simulink model "deteccao_erro_2014"  (R2014b)
settings: Solver=ode45  StartTime=72.6  StopTime=72.8  FixedStep=Ts  MaxStep=1e-7  RelTol=1e-5  AbsTol=1e-5
undefined symbols (not defined in the file or in its folder): C, L, sigbuilder_block, Ts
libraries: powerlib x59, dsparch4 x12, simulink x6, sps_avr x1, powerlib_meascontrol x1
(part 2 of 2)

== system deteccao_erro_2014/EHA1/DSP/Subsystem ==
  Vabc' : Inport
  Iabc_L : Inport  Port=2
  Demux : Demux  Outputs=3
  Demux6 : Demux  Outputs=3
  Gain1 : Gain  Gain=sqrt(2/3)
  Gain2 : Gain  Gain=sqrt(2/3)
  Gain3 : Gain  Gain=[1/sqrt(2), 1/sqrt(2), 1/sqrt(2); 1, -1/2, -1/2; 0, sqrt(3)/2, -sqrt(3)/2]  Multiplication=Matrix(K*u)
  Gain4 : Gain  Gain=[1/sqrt(2), 1/sqrt(2), 1/sqrt(2); 1, -1/2, -1/2; 0, sqrt(3)/2, -sqrt(3)/2]  Multiplication=Matrix(K*u)
  Scope15 : Scope  NumInputPorts=2
      settings: YMin=-600~-200  YMax=400~200  SaveName=ScopeData33
  Terminator : Terminator
  Terminator1 : Terminator
  Valpha' : Outport
  Vbeta' : Outport  Port=2
  Ialpha : Outport  Port=3
  Ibeta : Outport  Port=4
  wires:
  Gain1/1 -> Gain3/1
  Gain2/1 -> Gain4/1
  Gain3/1 -> Demux/1, Scope15/1  "Valphabeta0"
  Demux/2 -> Valpha'/1  "Valpha"
  Demux6/2 -> Ialpha/1  "Ialpha"
  Demux/3 -> Vbeta'/1  "Vbeta"
  Demux6/3 -> Ibeta/1  "Ibeta"
  Iabc_L/1 -> Gain2/1
  Vabc'/1 -> Gain1/1
  Gain4/1 -> Demux6/1, Scope15/2  "Ialphabeta0"
  Demux6/1 -> Terminator/1  "I0"
  Demux/1 -> Terminator1/1  "V0"

== system deteccao_erro_2014/EHA1/DSP/Subsystem1 ==
  Valpha' : Inport
  Vbeta' : Inport  Port=2
  Ialpha : Inport  Port=3
  Ibeta : Inport  Port=4
  Add : Sum
  Add10 : Sum
  Add3 : Sum  Inputs=+-
  Add4 : Sum  Inputs=+-
  LPF : dsparch4/Analog Filter Design  method=Butterworth  filttype=Lowpass  N=5  Wlo=2*pi*200  Whi=80  Rp=2  Rs=40
  Product{5..8} (4 alike) : Product
  Scope18 : Scope  NumInputPorts=4
      settings: TimeRange=0.015  YMin=120~175.6~-2050~-2100  YMax=250~177.8~-1400~-1400  SaveName=ScopeData35
  Posc : Outport
  q : Outport  Port=2
  wires:
  Product5/1 -> Add/1
  Product6/1 -> Add/2
  Add/1 -> Add4/2, LPF/1, Scope18/1  "P"
  Product7/1 -> Add3/1
  Product8/1 -> Add3/2
  Add3/1 -> q/1  "q"
  LPF/1 -> Add4/1, Scope18/2  "Pbarra"
  Vbeta'/1 -> Product7/1, Product6/1
  Ialpha/1 -> Product7/2, Product5/2
  Valpha'/1 -> Product8/1, Product5/1
  Ibeta/1 -> Product8/2, Product6/2
  Add10/1 -> Posc/1, Scope18/4  "Posc"
  Add4/1 -> Add10/2  "-Ptil"
  [Ploss1] -> Scope18/3, Add10/1  "Ploss"

== system deteccao_erro_2014/EHA1/DSP/Subsystem2 ==
  Valpha' : Inport
  Vbeta' : Inport  Port=2
  Posc : Inport  Port=3
  q : Inport  Port=4
  Add8 : Sum
  Add9 : Sum  Inputs=+-
  Divide{1..4} (4 alike) : Product  Inputs=***
  Fcn : Fcn  Expr=1/(u(1)^2+u(2)^2)
  Gain : Gain
  Gain5 : Gain  Gain=-1
  Mux : Mux  Inputs=2
  Scope20 : Scope  NumInputPorts=2
      settings: YMin=-8~-1e+12  YMax=8~2e+12  SaveName=ScopeData37
  Ialpha_p : Outport
  Ibeta_p : Outport  Port=2
  wires:
  Mux/1 -> Fcn/1
  Valpha'/1 -> Divide4/1, Mux/1, Divide1/1
  Vbeta'/1 -> Mux/2, Divide2/1, Divide3/1
  Posc/1 -> Gain5/1
  Fcn/1 -> Divide4/3, Divide3/3, Divide2/3, Divide1/3
  q/1 -> Gain/1
  Divide1/1 -> Add8/1
  Divide2/1 -> Add8/2
  Divide3/1 -> Add9/1
  Divide4/1 -> Add9/2
  Add9/1 -> Ibeta_p/1, Scope20/2  "Ibeta^*"
  Add8/1 -> Ialpha_p/1, Scope20/1  "Iaplha^*"
  Gain/1 -> Divide2/2, Divide4/2
  Gain5/1 -> Divide1/2, Divide3/2

== system deteccao_erro_2014/EHA1/DSP/Subsystem3 ==
  Ialpha_p : Inport
  Ibeta_p : Inport  Port=2
  Fcn1 : Fcn  Expr=sqrt(2/3)*u(1)
  Fcn2 : Fcn  Expr=sqrt(2/3)*(-1/2*u(1)+sqrt(3)/2*u(2))
  Fcn3 : Fcn  Expr=sqrt(2/3)*(-1/2*u(1)-sqrt(3)/2*u(2))
  Mux2 : Mux  Inputs=2
  Mux3 : Mux  Inputs=2
  Mux5 : Mux  Inputs=2
  Scope14 : Scope  NumInputPorts=3
      settings: TimeRange=0.08  YMin=-4~-4.5~-2  YMax=4.5~4~4.5  SaveName=ScopeData32
  Ia_C : Outport
  Ib_C : Outport  Port=2
  Ic_C : Outport  Port=3
  wires:
  Ibeta_p/1 -> Mux2/2, Mux3/2, Mux5/2
  Ialpha_p/1 -> Mux5/1, Mux2/1, Mux3/1
  Mux2/1 -> Fcn1/1
  Fcn1/1 -> Ia_C/1, Scope14/1  "Ia_C"
  Mux3/1 -> Fcn2/1
  Fcn2/1 -> Ib_C/1, Scope14/2  "Ib_C"
  Mux5/1 -> Fcn3/1
  Fcn3/1 -> Scope14/3, Ic_C/1  "Ic_C"

== system deteccao_erro_2014/EHA1/DSP/TCT ==
  Va : Inport
  Vb : Inport  Port=2
  Vc : Inport  Port=3
  Demux7 : Demux  Outputs=3
  Gain1 : Gain  Gain=sqrt(2/3)
  Gain3 : Gain  Gain=[1/sqrt(2), 1/sqrt(2), 1/sqrt(2); 1, -1/2, -1/2; 0, sqrt(3)/2, -sqrt(3)/2]  Multiplication=Matrix(K*u)
  Mux2 : Mux  Inputs=3
  valpha : Outport
  vbeta : Outport  Port=2
  wires:
  Gain3/1 -> Demux7/1  "Valphabeta0"
  Gain1/1 -> Gain3/1
  Mux2/1 -> Gain1/1
  Va/1 -> Mux2/1
  Vb/1 -> Mux2/2
  Vc/1 -> Mux2/3
  Demux7/2 -> valpha/1
  Demux7/3 -> vbeta/1

== system deteccao_erro_2014/EHA1/DSP/Transformada Inversa de Clarke ==
  valpha' : Inport
  vbeta' : Inport  Port=2
  Demux6 : Demux  Outputs=3
  Fcn10 : Fcn  Expr=sqrt(2/3)*(-1/2*u(1)+sqrt(3)/2*u(2))
  Fcn11 : Fcn  Expr=sqrt(2/3)*(-1/2*u(1)-sqrt(3)/2*u(2))
  Fcn9 : Fcn  Expr=sqrt(2/3)*(u(1) + 0*u(2))
  Mux{3,5,8..9} (4 alike) : Mux  Inputs=2
  Scope23 : Scope  NumInputPorts=3
      settings: YMin=-200~-200~-200  YMax=200~200~200  SaveName=ScopeData28
  va' : Outport
  vb' : Outport  Port=2
  vc' : Outport  Port=3
  wires:
  Fcn10/1 -> vb'/1, Scope23/2  "vb'"
  Demux6/1 -> Mux9/1
  valpha'/1 -> Mux5/1, Mux8/1, Mux3/1
  vbeta'/1 -> Mux3/2, Mux5/2, Mux8/2
  Mux5/1 -> Fcn10/1
  Mux3/1 -> Fcn9/1
  Fcn11/1 -> vc'/1, Scope23/3  "vc'"
  Fcn9/1 -> va'/1, Mux9/2  "va'"
  Mux8/1 -> Fcn11/1
  [Vabc_S] -> Demux6/1
  Mux9/1 -> Scope23/1

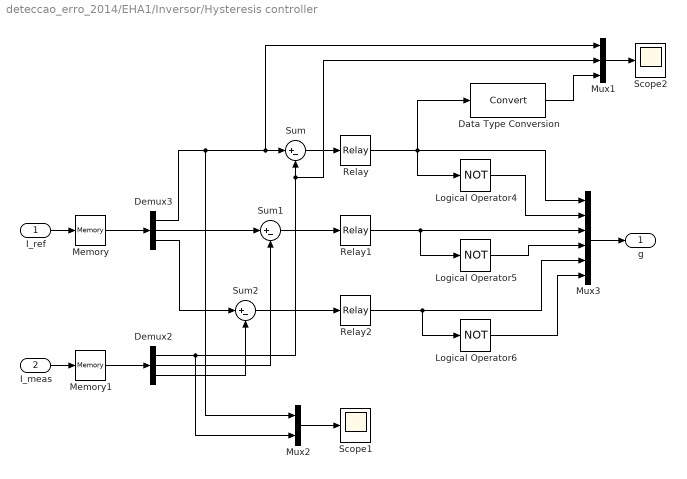
== system deteccao_erro_2014/EHA1/Inversor/Hysteresis controller ==
  I_ref : Inport
  I_meas : Inport  Port=2
  Data Type Conversion : DataTypeConversion
  Demux2 : Demux  Outputs=3
  Demux3 : Demux  Outputs=3
  Logical Operator4 : Logic  Operator=NOT  AllPortsSameDT=off  OutDataTypeStr=boolean
  Logical Operator5 : Logic  Operator=NOT  AllPortsSameDT=off  OutDataTypeStr=boolean
  Logical Operator6 : Logic  Operator=NOT  AllPortsSameDT=off  OutDataTypeStr=boolean
  Memory : Memory
  Memory1 : Memory
  Mux1 : Mux  Inputs=3
  Mux2 : Mux  Inputs=2
  Mux3 : Mux  Inputs=6
  Relay : Relay  OnSwitchValue=0.05  OffSwitchValue=-0.05  OutDataTypeStr=Inherit: Inherit via back propagation
  Relay1 : Relay  OnSwitchValue=0.05  OffSwitchValue=-0.05  OutDataTypeStr=Inherit: Inherit via back propagation
  Relay2 : Relay  OnSwitchValue=0.05  OffSwitchValue=-0.05  OutDataTypeStr=Inherit: Inherit via back propagation
  Scope1 : Scope
      settings: YMin=-3.75e+12  YMax=2.5e+11  SaveName=ScopeData30
  Scope2 : Scope
      settings: YMin=-4.5  YMax=5.5  SaveName=ScopeData6
  Sum : Sum  Inputs=|+-
  Sum1 : Sum  Inputs=|+-
  Sum2 : Sum  Inputs=|+-
  g : Outport
  wires:
  I_ref/1 -> Memory/1
  I_meas/1 -> Memory1/1
  Relay1/1 -> Logical Operator5/1, Mux3/3
  Demux3/1 -> Mux1/1, Sum/1, Mux2/1
  Logical Operator4/1 -> Mux3/2
  Logical Operator5/1 -> Mux3/4
  Logical Operator6/1 -> Mux3/6
  Mux3/1 -> g/1
  Demux2/1 -> Mux2/2, Mux1/2, Sum/2
  Memory/1 -> Demux3/1
  Memory1/1 -> Demux2/1
  Mux2/1 -> Scope1/1
  Sum/1 -> Relay/1
  Relay/1 -> Data Type Conversion/1, Mux3/1, Logical Operator4/1
  Demux3/2 -> Sum1/1
  Demux2/2 -> Sum1/2
  Sum1/1 -> Relay1/1
  Demux3/3 -> Sum2/1
  Sum2/1 -> Relay2/1
  Demux2/3 -> Sum2/2
  Relay2/1 -> Mux3/5, Logical Operator6/1
  Mux1/1 -> Scope2/1
  Data Type Conversion/1 -> Mux1/3

== system deteccao_erro_2014/EHA1/Inversor/PI controller ==
  Vdc : Inport
  Constant : Constant  Value=620
  LPF : dsparch4/Analog Filter Design  method=Butterworth  filttype=Lowpass  N=5  Wlo=2*pi*200  Whi=80  Rp=2  Rs=40
  PID Controller : simulink/Continuous/PID Controller  Controller=PI  TimeDomain=Continuous-time  SampleTime=-1  IntegratorMethod=Forward Euler  FilterMethod=Forward Euler  Form=Parallel  P=5  I=7  D=0  N=100  InitialConditionSource=internal  InitialConditionForIntegrator=0  InitialConditionForFilter=0  ExternalReset=none  LimitOutput=off  UpperSaturationLimit=inf  LowerSaturationLimit=-inf  LinearizeAsGain=on  AntiWindupMode=none  Kb=1  TrackingMode=off  Kt=1  PParamMin=[]  PParamMax=[]  IParamMin=[]  IParamMax=[]  DParamMin=[]  DParamMax=[]  NParamMin=[]  NParamMax=[]  KbParamMin=[]  KbParamMax=[]  KtParamMin=[]  KtParamMax=[]  POutMin=[]  POutMax=[]  IOutMin=[]  IOutMax=[]  DOutMin=[]  DOutMax=[]  NOutMin=[]  NOutMax=[]  KbOutMin=[]  KbOutMax=[]  KtOutMin=[]  KtOutMax=[]  IntegratorOutMin=[]  IntegratorOutMax=[]  FilterOutMin=[]  FilterOutMax=[]  SumOutMin=[]  SumOutMax=[]  SumI1OutMin=[]  SumI1OutMax=[]  SumI2OutMin=[]  SumI2OutMax=[]  SumI3OutMin=[]  SumI3OutMax=[]  SumDOutMin=[]  SumDOutMax=[]  SaturationOutMin=[]  SaturationOutMax=[]  IntegratorContinuousStateAttributes=''  IntegratorStateMustResolveToSignalObject=off  IntegratorRTWStateStorageClass=Auto  FilterContinuousStateAttributes=''  FilterStateMustResolveToSignalObject=off  FilterRTWStateStorageClass=Auto  DifferentiatorICPrevScaledInput=0  DifferentiatorOutMin=[]  DifferentiatorOutMax=[]  UseFilter=on
  Scope : Scope  NumInputPorts=3
      settings: TimeRange=0.015  YMin=-5~-5~-5  YMax=5~5~5  SaveName=ScopeData18
  Signal Builder : Subsystem  Tag=STV Subsys  LoadFcn=sigbuilder_block('load');  StartFcn=sigbuilder_block('start');  StopFcn=sigbuilder_block('stop');  ClipboardFcn=sigbuilder_block('clipboard');  mask(Sigbuilder block){}
      mask help: Simulink:masks:SigbuilderBlock_MD
      mask init:
      | if ~strcmp(get_param(bdroot(gcbh),'SimulationStatus'),'stopped') tuvar = sigbuilder_block('maskInit'); end
      settings: CopyFcn=sigbuilder_block('copy');  DeleteFcn=sigbuilder_block('delete');  ModelCloseFcn=sigbuilder_block('modelClose');  PreSaveFcn=sigbuilder_block('preSave');  PauseFcn=sigbuilder_block('pause');  ContinueFcn=sigbuilder_block('continue');  NameChangeFcn=sigbuilder_block('namechange');  OpenFcn=sigbuilder_block('open',[437.6 199.2 550.4 400 ]);  CloseFcn=sigbuilder_block('close');
      mask Display: plot(0, 0, 100, 100,[2, 2, 32, 32, 2], [68, 8, 8, 68, 68],[32, 2], [38, 38], [32, 19, 2],[53, 60, 44], [32, 17, 17, 2],[16, 16, 31, 31]);txt = getActiveGroup(gcbh);text(2, 100, txt,'verticalAlignment', 'top');
  Sum : Sum  Inputs=|-+
  Ploss : Outport
  wires:
  Vdc/1 -> Scope/1, Sum/1  "Vdc"
  Sum/1 -> LPF/1, Scope/2  "Vdc-step"
  PID Controller/1 -> Scope/3, Ploss/1  "Ploss"
  LPF/1 -> PID Controller/1
  Signal Builder/1(Signal 2) -> Sum/2

== system deteccao_erro_2014/EHA2/DSP/Calculo de potência Instantânea ==
  Ialpha' : Inport
  Ibeta' : Inport  Port=2
  valpha : Inport  Port=3
  vbeta : Inport  Port=4
  Fcn5 : Fcn  Expr=u(1)*u(3)+u(2)*u(4)
  Fcn6 : Fcn  Expr=u(2)*u(3)-u(1)*u(4)
  LPF : dsparch4/Analog Filter Design  method=Butterworth  filttype=Lowpass  N=5  Wlo=2*pi*100  Whi=80  Rp=2  Rs=40
  LPF1 : dsparch4/Analog Filter Design  method=Butterworth  filttype=Lowpass  N=5  Wlo=2*pi*100  Whi=80  Rp=2  Rs=40
  Mux2 : Mux
  pbarra' : Outport
  qbarra' : Outport  Port=2
  wires:
  Ibeta'/1 -> Mux2/4
  Ialpha'/1 -> Mux2/3
  LPF1/1 -> qbarra'/1
  LPF/1 -> pbarra'/1
  Mux2/1 -> Fcn6/1, Fcn5/1
  Fcn6/1 -> LPF1/1  "q'"
  Fcn5/1 -> LPF/1  "p'"
  vbeta/1 -> Mux2/2
  valpha/1 -> Mux2/1

== system deteccao_erro_2014/EHA2/DSP/Cálculo de tensões alpha-beta ==
  Ialpha' : Inport
  Ibeta' : Inport  Port=2
  pbarra' : Inport  Port=3
  qbarra' : Inport  Port=4
  Add8 : Sum
  Divide5 : Product  Inputs=**
  Divide6 : Product  Inputs=**
  Divide8 : Product  Inputs=*/
  Divide9 : Product  Inputs=*/
  Fcn7 : Fcn  Expr=u(3)*u(1)-u(4)*u(2)
  Fcn8 : Fcn  Expr=u(4)*u(1)+u(3)*u(2)
  Gain8 : Gain
  Gain9 : Gain
  Mux6 : Mux
  valpha' : Outport
  vbeta' : Outport  Port=2
  wires:
  pbarra'/1 -> Gain8/1
  Divide5/1 -> Add8/1
  Divide6/1 -> Add8/2
  Gain8/1 -> Mux6/1
  Fcn8/1 -> Divide9/1
  Mux6/1 -> Fcn8/1, Fcn7/1
  qbarra'/1 -> Gain9/1
  Divide8/1 -> valpha'/1
  Fcn7/1 -> Divide8/1
  Gain9/1 -> Mux6/2
  Divide9/1 -> vbeta'/1
  Ibeta'/1 -> Mux6/4, Divide6/1, Divide6/2
  Ialpha'/1 -> Mux6/3, Divide5/1, Divide5/2
  Add8/1 -> Divide9/2, Divide8/2

== system deteccao_erro_2014/EHA2/DSP/PLL ==
  Va : Inport
  Vb : Inport  Port=2
  Vc : Inport  Port=3
  Add10 : Sum
  Add3 : Sum  Inputs=+-
  Add4 : Sum  Inputs=+-
  Fcn1 : Fcn  Expr=sin(u(1))
  Fcn2 : Fcn  Expr=sin(u(1)+2*pi/3)
  Fcn3 : Fcn  Expr=sin(u(1)-pi/2)
  Fcn4 : Fcn  Expr=-cos(u(1)-pi/2)
  Integrator : Integrator
  PID Controller : simulink/Continuous/PID Controller  Controller=PI  TimeDomain=Continuous-time  SampleTime=-1  IntegratorMethod=Forward Euler  FilterMethod=Forward Euler  Form=Parallel  P=30  I=1  D=0  N=100  InitialConditionSource=internal  InitialConditionForIntegrator=0  InitialConditionForFilter=0  ExternalReset=none  LimitOutput=off  UpperSaturationLimit=inf  LowerSaturationLimit=-inf  LinearizeAsGain=on  AntiWindupMode=none  Kb=1  TrackingMode=off  Kt=1  PParamMin=[]  PParamMax=[]  IParamMin=[]  IParamMax=[]  DParamMin=[]  DParamMax=[]  NParamMin=[]  NParamMax=[]  KbParamMin=[]  KbParamMax=[]  KtParamMin=[]  KtParamMax=[]  POutMin=[]  POutMax=[]  IOutMin=[]  IOutMax=[]  DOutMin=[]  DOutMax=[]  NOutMin=[]  NOutMax=[]  KbOutMin=[]  KbOutMax=[]  KtOutMin=[]  KtOutMax=[]  IntegratorOutMin=[]  IntegratorOutMax=[]  FilterOutMin=[]  FilterOutMax=[]  SumOutMin=[]  SumOutMax=[]  SumI1OutMin=[]  SumI1OutMax=[]  SumI2OutMin=[]  SumI2OutMax=[]  SumI3OutMin=[]  SumI3OutMax=[]  SumDOutMin=[]  SumDOutMax=[]  SaturationOutMin=[]  SaturationOutMax=[]  IntegratorContinuousStateAttributes=''  IntegratorStateMustResolveToSignalObject=off  IntegratorRTWStateStorageClass=Auto  FilterContinuousStateAttributes=''  FilterStateMustResolveToSignalObject=off  FilterRTWStateStorageClass=Auto  DifferentiatorICPrevScaledInput=0  DifferentiatorOutMin=[]  DifferentiatorOutMax=[]  UseFilter=on
  Product5 : Product
  Product6 : Product
  Ialpha' : Outport
  Ibeta' : Outport  Port=2
  wires:
  Va/1 -> Add3/1
  Add3/1 -> Product5/2  "Vab"
  Vc/1 -> Add4/1
  Fcn3/1 -> Ialpha'/1
  Fcn1/1 -> Product5/1
  Fcn2/1 -> Product6/2
  Integrator/1 -> Fcn2/1, Fcn4/1, Fcn1/1, Fcn3/1  "wt"
  Product6/1 -> Add10/2
  Vb/1 -> Add4/2, Add3/2
  Product5/1 -> Add10/1
  Add4/1 -> Product6/1  "Vcb"
  PID Controller/1 -> Integrator/1  "w"
  Add10/1 -> PID Controller/1  "P3phi"
  Fcn4/1 -> Ibeta'/1

== system deteccao_erro_2014/EHA2/DSP/Subsystem ==
  Vabc' : Inport
  Iabc_L : Inport  Port=2
  Demux : Demux  Outputs=3
  Demux6 : Demux  Outputs=3
  Gain1 : Gain  Gain=sqrt(2/3)
  Gain2 : Gain  Gain=sqrt(2/3)
  Gain3 : Gain  Gain=[1/sqrt(2), 1/sqrt(2), 1/sqrt(2); 1, -1/2, -1/2; 0, sqrt(3)/2, -sqrt(3)/2]  Multiplication=Matrix(K*u)
  Gain4 : Gain  Gain=[1/sqrt(2), 1/sqrt(2), 1/sqrt(2); 1, -1/2, -1/2; 0, sqrt(3)/2, -sqrt(3)/2]  Multiplication=Matrix(K*u)
  Scope15 : Scope  NumInputPorts=2
      settings: YMin=-600~-200  YMax=400~200  SaveName=ScopeData33
  Terminator : Terminator
  Terminator1 : Terminator
  Valpha' : Outport
  Vbeta' : Outport  Port=2
  Ialpha : Outport  Port=3
  Ibeta : Outport  Port=4
  wires:
  Gain1/1 -> Gain3/1
  Gain2/1 -> Gain4/1
  Gain3/1 -> Demux/1, Scope15/1  "Valphabeta0"
  Demux/2 -> Valpha'/1  "Valpha"
  Demux6/2 -> Ialpha/1  "Ialpha"
  Demux/3 -> Vbeta'/1  "Vbeta"
  Demux6/3 -> Ibeta/1  "Ibeta"
  Iabc_L/1 -> Gain2/1
  Vabc'/1 -> Gain1/1
  Gain4/1 -> Demux6/1, Scope15/2  "Ialphabeta0"
  Demux6/1 -> Terminator/1  "I0"
  Demux/1 -> Terminator1/1  "V0"

== system deteccao_erro_2014/EHA2/DSP/Subsystem1 ==
  Valpha' : Inport
  Vbeta' : Inport  Port=2
  Ialpha : Inport  Port=3
  Ibeta : Inport  Port=4
  Add : Sum
  Add10 : Sum
  Add3 : Sum  Inputs=+-
  Add4 : Sum  Inputs=+-
  LPF : dsparch4/Analog Filter Design  method=Butterworth  filttype=Lowpass  N=5  Wlo=2*pi*200  Whi=80  Rp=2  Rs=40
  Product{5..8} (4 alike) : Product
  Scope18 : Scope  NumInputPorts=4
      settings: TimeRange=0.015  YMin=24750~27050~-494~-2500  YMax=29750~27900~-478~2000  SaveName=ScopeData35
  Posc : Outport
  q : Outport  Port=2
  wires:
  Product5/1 -> Add/1
  Product6/1 -> Add/2
  Add/1 -> Add4/2, LPF/1, Scope18/1  "P"
  Product7/1 -> Add3/1
  Product8/1 -> Add3/2
  Add3/1 -> q/1  "q"
  LPF/1 -> Add4/1, Scope18/2  "Pbarra"
  Vbeta'/1 -> Product7/1, Product6/1
  Ialpha/1 -> Product7/2, Product5/2
  Valpha'/1 -> Product8/1, Product5/1
  Ibeta/1 -> Product8/2, Product6/2
  Add10/1 -> Posc/1, Scope18/4  "Posc"
  Add4/1 -> Add10/2  "-Ptil"
  [Ploss2] -> Scope18/3, Add10/1  "Ploss"

== system deteccao_erro_2014/EHA2/DSP/Subsystem2 ==
  Valpha' : Inport
  Vbeta' : Inport  Port=2
  Posc : Inport  Port=3
  q : Inport  Port=4
  Add8 : Sum
  Add9 : Sum  Inputs=+-
  Divide{1..4} (4 alike) : Product  Inputs=***
  Fcn : Fcn  Expr=1/(u(1)^2+u(2)^2)
  Gain : Gain
  Gain5 : Gain  Gain=-1
  Mux : Mux  Inputs=2
  Scope20 : Scope  NumInputPorts=2
      settings: YMin=-8~-1e+12  YMax=8~2e+12  SaveName=ScopeData37
  Ialpha_p : Outport
  Ibeta_p : Outport  Port=2
  wires:
  Mux/1 -> Fcn/1
  Valpha'/1 -> Divide4/1, Mux/1, Divide1/1
  Vbeta'/1 -> Mux/2, Divide2/1, Divide3/1
  Posc/1 -> Gain5/1
  Fcn/1 -> Divide4/3, Divide3/3, Divide2/3, Divide1/3
  q/1 -> Gain/1
  Divide1/1 -> Add8/1
  Divide2/1 -> Add8/2
  Divide3/1 -> Add9/1
  Divide4/1 -> Add9/2
  Add9/1 -> Ibeta_p/1, Scope20/2  "Ibeta^*"
  Add8/1 -> Ialpha_p/1, Scope20/1  "Iaplha^*"
  Gain/1 -> Divide2/2, Divide4/2
  Gain5/1 -> Divide1/2, Divide3/2

== system deteccao_erro_2014/EHA2/DSP/Subsystem3 ==
  Ialpha_p : Inport
  Ibeta_p : Inport  Port=2
  Fcn1 : Fcn  Expr=sqrt(2/3)*u(1)
  Fcn2 : Fcn  Expr=sqrt(2/3)*(-1/2*u(1)+sqrt(3)/2*u(2))
  Fcn3 : Fcn  Expr=sqrt(2/3)*(-1/2*u(1)-sqrt(3)/2*u(2))
  Mux2 : Mux  Inputs=2
  Mux3 : Mux  Inputs=2
  Mux5 : Mux  Inputs=2
  Scope14 : Scope  NumInputPorts=3
      settings: TimeRange=0.08  YMin=-4~-4.5~-2  YMax=4.5~4~4.5  SaveName=ScopeData32
  Ia_C : Outport
  Ib_C : Outport  Port=2
  Ic_C : Outport  Port=3
  wires:
  Ibeta_p/1 -> Mux2/2, Mux3/2, Mux5/2
  Ialpha_p/1 -> Mux5/1, Mux2/1, Mux3/1
  Mux2/1 -> Fcn1/1
  Fcn1/1 -> Ia_C/1, Scope14/1  "Ia_C"
  Mux3/1 -> Fcn2/1
  Fcn2/1 -> Ib_C/1, Scope14/2  "Ib_C"
  Mux5/1 -> Fcn3/1
  Fcn3/1 -> Scope14/3, Ic_C/1  "Ic_C"

== system deteccao_erro_2014/EHA2/DSP/TCT ==
  Va : Inport
  Vb : Inport  Port=2
  Vc : Inport  Port=3
  Demux7 : Demux  Outputs=3
  Gain1 : Gain  Gain=sqrt(2/3)
  Gain3 : Gain  Gain=[1/sqrt(2), 1/sqrt(2), 1/sqrt(2); 1, -1/2, -1/2; 0, sqrt(3)/2, -sqrt(3)/2]  Multiplication=Matrix(K*u)
  Mux2 : Mux  Inputs=3
  valpha : Outport
  vbeta : Outport  Port=2
  wires:
  Gain3/1 -> Demux7/1  "Valphabeta0"
  Gain1/1 -> Gain3/1
  Mux2/1 -> Gain1/1
  Va/1 -> Mux2/1
  Vb/1 -> Mux2/2
  Vc/1 -> Mux2/3
  Demux7/2 -> valpha/1
  Demux7/3 -> vbeta/1

== system deteccao_erro_2014/EHA2/DSP/Transformada Inversa de Clarke ==
  valpha' : Inport
  vbeta' : Inport  Port=2
  Demux6 : Demux  Outputs=3
  Fcn10 : Fcn  Expr=sqrt(2/3)*(-1/2*u(1)+sqrt(3)/2*u(2))
  Fcn11 : Fcn  Expr=sqrt(2/3)*(-1/2*u(1)-sqrt(3)/2*u(2))
  Fcn9 : Fcn  Expr=sqrt(2/3)*(u(1) + 0*u(2))
  Mux{3,5,8..9} (4 alike) : Mux  Inputs=2
  Scope23 : Scope  NumInputPorts=3
      settings: YMin=-200~-200~-200  YMax=200~200~200  SaveName=ScopeData28
  va' : Outport
  vb' : Outport  Port=2
  vc' : Outport  Port=3
  wires:
  Fcn10/1 -> vb'/1, Scope23/2  "vb'"
  Demux6/1 -> Mux9/1
  valpha'/1 -> Mux5/1, Mux8/1, Mux3/1
  vbeta'/1 -> Mux3/2, Mux5/2, Mux8/2
  Mux5/1 -> Fcn10/1
  Mux3/1 -> Fcn9/1
  Fcn11/1 -> vc'/1, Scope23/3  "vc'"
  Fcn9/1 -> va'/1, Mux9/2  "va'"
  Mux8/1 -> Fcn11/1
  [Vabc_S] -> Demux6/1
  Mux9/1 -> Scope23/1

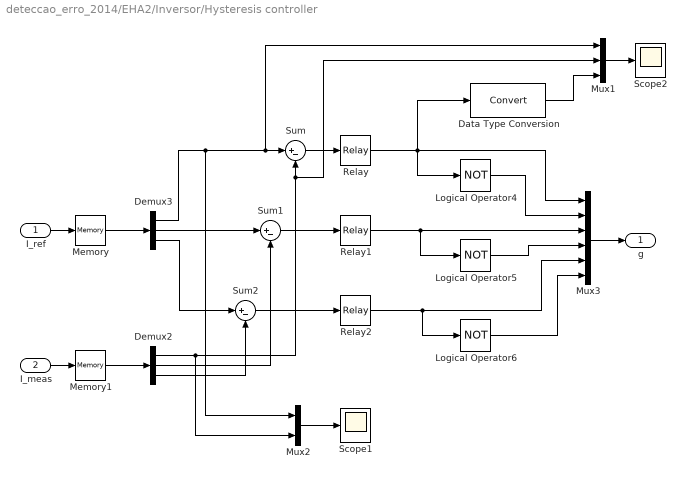
== system deteccao_erro_2014/EHA2/Inversor/Hysteresis controller ==
  I_ref : Inport
  I_meas : Inport  Port=2
  Data Type Conversion : DataTypeConversion
  Demux2 : Demux  Outputs=3
  Demux3 : Demux  Outputs=3
  Logical Operator4 : Logic  Operator=NOT  AllPortsSameDT=off  OutDataTypeStr=boolean
  Logical Operator5 : Logic  Operator=NOT  AllPortsSameDT=off  OutDataTypeStr=boolean
  Logical Operator6 : Logic  Operator=NOT  AllPortsSameDT=off  OutDataTypeStr=boolean
  Memory : Memory
  Memory1 : Memory
  Mux1 : Mux  Inputs=3
  Mux2 : Mux  Inputs=2
  Mux3 : Mux  Inputs=6
  Relay : Relay  OnSwitchValue=0.05  OffSwitchValue=-0.05  OutDataTypeStr=Inherit: Inherit via back propagation
  Relay1 : Relay  OnSwitchValue=0.05  OffSwitchValue=-0.05  OutDataTypeStr=Inherit: Inherit via back propagation
  Relay2 : Relay  OnSwitchValue=0.05  OffSwitchValue=-0.05  OutDataTypeStr=Inherit: Inherit via back propagation
  Scope1 : Scope
      settings: YMin=-3.75e+12  YMax=2.5e+11  SaveName=ScopeData30
  Scope2 : Scope
      settings: YMin=-4.5  YMax=5.5  SaveName=ScopeData6
  Sum : Sum  Inputs=|+-
  Sum1 : Sum  Inputs=|+-
  Sum2 : Sum  Inputs=|+-
  g : Outport
  wires:
  I_ref/1 -> Memory/1
  I_meas/1 -> Memory1/1
  Relay1/1 -> Logical Operator5/1, Mux3/3
  Demux3/1 -> Mux1/1, Sum/1, Mux2/1
  Logical Operator4/1 -> Mux3/2
  Logical Operator5/1 -> Mux3/4
  Logical Operator6/1 -> Mux3/6
  Mux3/1 -> g/1
  Demux2/1 -> Mux2/2, Mux1/2, Sum/2
  Memory/1 -> Demux3/1
  Memory1/1 -> Demux2/1
  Mux2/1 -> Scope1/1
  Sum/1 -> Relay/1
  Relay/1 -> Data Type Conversion/1, Mux3/1, Logical Operator4/1
  Demux3/2 -> Sum1/1
  Demux2/2 -> Sum1/2
  Sum1/1 -> Relay1/1
  Demux3/3 -> Sum2/1
  Sum2/1 -> Relay2/1
  Demux2/3 -> Sum2/2
  Relay2/1 -> Mux3/5, Logical Operator6/1
  Mux1/1 -> Scope2/1
  Data Type Conversion/1 -> Mux1/3

== system deteccao_erro_2014/EHA2/Inversor/PI controller ==
  Vdc : Inport
  Constant : Constant  Value=480
  LPF : dsparch4/Analog Filter Design  method=Butterworth  filttype=Lowpass  N=5  Wlo=2*pi*200  Whi=80  Rp=2  Rs=40
  PID Controller : simulink/Continuous/PID Controller  Controller=PI  TimeDomain=Continuous-time  SampleTime=-1  IntegratorMethod=Forward Euler  FilterMethod=Forward Euler  Form=Parallel  P=5  I=7  D=0  N=100  InitialConditionSource=internal  InitialConditionForIntegrator=0  InitialConditionForFilter=0  ExternalReset=none  LimitOutput=off  UpperSaturationLimit=inf  LowerSaturationLimit=-inf  LinearizeAsGain=on  AntiWindupMode=none  Kb=1  TrackingMode=off  Kt=1  PParamMin=[]  PParamMax=[]  IParamMin=[]  IParamMax=[]  DParamMin=[]  DParamMax=[]  NParamMin=[]  NParamMax=[]  KbParamMin=[]  KbParamMax=[]  KtParamMin=[]  KtParamMax=[]  POutMin=[]  POutMax=[]  IOutMin=[]  IOutMax=[]  DOutMin=[]  DOutMax=[]  NOutMin=[]  NOutMax=[]  KbOutMin=[]  KbOutMax=[]  KtOutMin=[]  KtOutMax=[]  IntegratorOutMin=[]  IntegratorOutMax=[]  FilterOutMin=[]  FilterOutMax=[]  SumOutMin=[]  SumOutMax=[]  SumI1OutMin=[]  SumI1OutMax=[]  SumI2OutMin=[]  SumI2OutMax=[]  SumI3OutMin=[]  SumI3OutMax=[]  SumDOutMin=[]  SumDOutMax=[]  SaturationOutMin=[]  SaturationOutMax=[]  IntegratorContinuousStateAttributes=''  IntegratorStateMustResolveToSignalObject=off  IntegratorRTWStateStorageClass=Auto  FilterContinuousStateAttributes=''  FilterStateMustResolveToSignalObject=off  FilterRTWStateStorageClass=Auto  DifferentiatorICPrevScaledInput=0  DifferentiatorOutMin=[]  DifferentiatorOutMax=[]  UseFilter=on
  Scope : Scope  NumInputPorts=2
      settings: TimeRange=0.015  YMin=-550~450  YMax=25~1025  SaveName=ScopeData15
  Sum : Sum  Inputs=|-+
  Ploss : Outport
  wires:
  Vdc/1 -> Sum/1, Scope/2
  Sum/1 -> LPF/1, Scope/1
  Constant/1 -> Sum/2
  PID Controller/1 -> Ploss/1
  LPF/1 -> PID Controller/1

== system deteccao_erro_2014/EHA3/DSP/Calculo de potência Instantânea ==
  Ialpha' : Inport
  Ibeta' : Inport  Port=2
  valpha : Inport  Port=3
  vbeta : Inport  Port=4
  Fcn5 : Fcn  Expr=u(1)*u(3)+u(2)*u(4)
  Fcn6 : Fcn  Expr=u(2)*u(3)-u(1)*u(4)
  LPF : dsparch4/Analog Filter Design  method=Butterworth  filttype=Lowpass  N=5  Wlo=2*pi*100  Whi=80  Rp=2  Rs=40
  LPF1 : dsparch4/Analog Filter Design  method=Butterworth  filttype=Lowpass  N=5  Wlo=2*pi*100  Whi=80  Rp=2  Rs=40
  Mux2 : Mux
  pbarra' : Outport
  qbarra' : Outport  Port=2
  wires:
  Ibeta'/1 -> Mux2/4
  Ialpha'/1 -> Mux2/3
  LPF1/1 -> qbarra'/1
  LPF/1 -> pbarra'/1
  Mux2/1 -> Fcn6/1, Fcn5/1
  Fcn6/1 -> LPF1/1  "q'"
  Fcn5/1 -> LPF/1  "p'"
  vbeta/1 -> Mux2/2
  valpha/1 -> Mux2/1

== system deteccao_erro_2014/EHA3/DSP/Cálculo de tensões alpha-beta ==
  Ialpha' : Inport
  Ibeta' : Inport  Port=2
  pbarra' : Inport  Port=3
  qbarra' : Inport  Port=4
  Add8 : Sum
  Divide5 : Product  Inputs=**
  Divide6 : Product  Inputs=**
  Divide8 : Product  Inputs=*/
  Divide9 : Product  Inputs=*/
  Fcn7 : Fcn  Expr=u(3)*u(1)-u(4)*u(2)
  Fcn8 : Fcn  Expr=u(4)*u(1)+u(3)*u(2)
  Gain8 : Gain
  Gain9 : Gain
  Mux6 : Mux
  valpha' : Outport
  vbeta' : Outport  Port=2
  wires:
  pbarra'/1 -> Gain8/1
  Divide5/1 -> Add8/1
  Divide6/1 -> Add8/2
  Gain8/1 -> Mux6/1
  Fcn8/1 -> Divide9/1
  Mux6/1 -> Fcn8/1, Fcn7/1
  qbarra'/1 -> Gain9/1
  Divide8/1 -> valpha'/1
  Fcn7/1 -> Divide8/1
  Gain9/1 -> Mux6/2
  Divide9/1 -> vbeta'/1
  Ibeta'/1 -> Mux6/4, Divide6/1, Divide6/2
  Ialpha'/1 -> Mux6/3, Divide5/1, Divide5/2
  Add8/1 -> Divide9/2, Divide8/2

== system deteccao_erro_2014/EHA3/DSP/PLL ==
  Va : Inport
  Vb : Inport  Port=2
  Vc : Inport  Port=3
  Add10 : Sum
  Add3 : Sum  Inputs=+-
  Add4 : Sum  Inputs=+-
  Fcn1 : Fcn  Expr=sin(u(1))
  Fcn2 : Fcn  Expr=sin(u(1)+2*pi/3)
  Fcn3 : Fcn  Expr=sin(u(1)-pi/2)
  Fcn4 : Fcn  Expr=-cos(u(1)-pi/2)
  Integrator : Integrator
  PID Controller : simulink/Continuous/PID Controller  Controller=PI  TimeDomain=Continuous-time  SampleTime=-1  IntegratorMethod=Forward Euler  FilterMethod=Forward Euler  Form=Parallel  P=30  I=1  D=0  N=100  InitialConditionSource=internal  InitialConditionForIntegrator=0  InitialConditionForFilter=0  ExternalReset=none  LimitOutput=off  UpperSaturationLimit=inf  LowerSaturationLimit=-inf  LinearizeAsGain=on  AntiWindupMode=none  Kb=1  TrackingMode=off  Kt=1  PParamMin=[]  PParamMax=[]  IParamMin=[]  IParamMax=[]  DParamMin=[]  DParamMax=[]  NParamMin=[]  NParamMax=[]  KbParamMin=[]  KbParamMax=[]  KtParamMin=[]  KtParamMax=[]  POutMin=[]  POutMax=[]  IOutMin=[]  IOutMax=[]  DOutMin=[]  DOutMax=[]  NOutMin=[]  NOutMax=[]  KbOutMin=[]  KbOutMax=[]  KtOutMin=[]  KtOutMax=[]  IntegratorOutMin=[]  IntegratorOutMax=[]  FilterOutMin=[]  FilterOutMax=[]  SumOutMin=[]  SumOutMax=[]  SumI1OutMin=[]  SumI1OutMax=[]  SumI2OutMin=[]  SumI2OutMax=[]  SumI3OutMin=[]  SumI3OutMax=[]  SumDOutMin=[]  SumDOutMax=[]  SaturationOutMin=[]  SaturationOutMax=[]  IntegratorContinuousStateAttributes=''  IntegratorStateMustResolveToSignalObject=off  IntegratorRTWStateStorageClass=Auto  FilterContinuousStateAttributes=''  FilterStateMustResolveToSignalObject=off  FilterRTWStateStorageClass=Auto  DifferentiatorICPrevScaledInput=0  DifferentiatorOutMin=[]  DifferentiatorOutMax=[]  UseFilter=on
  Product5 : Product
  Product6 : Product
  Ialpha' : Outport
  Ibeta' : Outport  Port=2
  wires:
  Va/1 -> Add3/1
  Add3/1 -> Product5/2  "Vab"
  Vc/1 -> Add4/1
  Fcn3/1 -> Ialpha'/1
  Fcn1/1 -> Product5/1
  Fcn2/1 -> Product6/2
  Integrator/1 -> Fcn2/1, Fcn4/1, Fcn1/1, Fcn3/1  "wt"
  Product6/1 -> Add10/2
  Vb/1 -> Add4/2, Add3/2
  Product5/1 -> Add10/1
  Add4/1 -> Product6/1  "Vcb"
  PID Controller/1 -> Integrator/1  "w"
  Add10/1 -> PID Controller/1  "P3phi"
  Fcn4/1 -> Ibeta'/1

== system deteccao_erro_2014/EHA3/DSP/Subsystem ==
  Vabc' : Inport
  Iabc_L : Inport  Port=2
  Demux : Demux  Outputs=3
  Demux6 : Demux  Outputs=3
  Gain1 : Gain  Gain=sqrt(2/3)
  Gain2 : Gain  Gain=sqrt(2/3)
  Gain3 : Gain  Gain=[1/sqrt(2), 1/sqrt(2), 1/sqrt(2); 1, -1/2, -1/2; 0, sqrt(3)/2, -sqrt(3)/2]  Multiplication=Matrix(K*u)
  Gain4 : Gain  Gain=[1/sqrt(2), 1/sqrt(2), 1/sqrt(2); 1, -1/2, -1/2; 0, sqrt(3)/2, -sqrt(3)/2]  Multiplication=Matrix(K*u)
  Scope15 : Scope  NumInputPorts=2
      settings: YMin=-600~-200  YMax=400~200  SaveName=ScopeData33
  Terminator : Terminator
  Terminator1 : Terminator
  Valpha' : Outport
  Vbeta' : Outport  Port=2
  Ialpha : Outport  Port=3
  Ibeta : Outport  Port=4
  wires:
  Gain1/1 -> Gain3/1
  Gain2/1 -> Gain4/1
  Gain3/1 -> Demux/1, Scope15/1  "Valphabeta0"
  Demux/2 -> Valpha'/1  "Valpha"
  Demux6/2 -> Ialpha/1  "Ialpha"
  Demux/3 -> Vbeta'/1  "Vbeta"
  Demux6/3 -> Ibeta/1  "Ibeta"
  Iabc_L/1 -> Gain2/1
  Vabc'/1 -> Gain1/1
  Gain4/1 -> Demux6/1, Scope15/2  "Ialphabeta0"
  Demux6/1 -> Terminator/1  "I0"
  Demux/1 -> Terminator1/1  "V0"

== system deteccao_erro_2014/EHA3/DSP/Subsystem1 ==
  Valpha' : Inport
  Vbeta' : Inport  Port=2
  Ialpha : Inport  Port=3
  Ibeta : Inport  Port=4
  Add : Sum
  Add10 : Sum
  Add3 : Sum  Inputs=+-
  Add4 : Sum  Inputs=+-
  LPF : dsparch4/Analog Filter Design  method=Butterworth  filttype=Lowpass  N=5  Wlo=2*pi*200  Whi=80  Rp=2  Rs=40
  Product{5..8} (4 alike) : Product
  Scope18 : Scope  NumInputPorts=4
      settings: TimeRange=0.015  YMin=120~174.3~-1500~-1560  YMax=280~174.675~-1440~-1430  SaveName=ScopeData35
  Posc : Outport
  q : Outport  Port=2
  wires:
  Product5/1 -> Add/1
  Product6/1 -> Add/2
  Add/1 -> Add4/2, LPF/1, Scope18/1  "P"
  Product7/1 -> Add3/1
  Product8/1 -> Add3/2
  Add3/1 -> q/1  "q"
  LPF/1 -> Add4/1, Scope18/2  "Pbarra"
  Vbeta'/1 -> Product7/1, Product6/1
  Ialpha/1 -> Product7/2, Product5/2
  Valpha'/1 -> Product8/1, Product5/1
  Ibeta/1 -> Product8/2, Product6/2
  Add10/1 -> Posc/1, Scope18/4  "Posc"
  Add4/1 -> Add10/2  "-Ptil"
  [Ploss3] -> Scope18/3, Add10/1  "Ploss"

== system deteccao_erro_2014/EHA3/DSP/Subsystem2 ==
  Valpha' : Inport
  Vbeta' : Inport  Port=2
  Posc : Inport  Port=3
  q : Inport  Port=4
  Add8 : Sum
  Add9 : Sum  Inputs=+-
  Divide{1..4} (4 alike) : Product  Inputs=***
  Fcn : Fcn  Expr=1/(u(1)^2+u(2)^2)
  Gain : Gain
  Gain5 : Gain  Gain=-1
  Mux : Mux  Inputs=2
  Scope20 : Scope  NumInputPorts=2
      settings: YMin=-8~-1e+12  YMax=8~2e+12  SaveName=ScopeData37
  Ialpha_p : Outport
  Ibeta_p : Outport  Port=2
  wires:
  Mux/1 -> Fcn/1
  Valpha'/1 -> Divide4/1, Mux/1, Divide1/1
  Vbeta'/1 -> Mux/2, Divide2/1, Divide3/1
  Posc/1 -> Gain5/1
  Fcn/1 -> Divide4/3, Divide3/3, Divide2/3, Divide1/3
  q/1 -> Gain/1
  Divide1/1 -> Add8/1
  Divide2/1 -> Add8/2
  Divide3/1 -> Add9/1
  Divide4/1 -> Add9/2
  Add9/1 -> Ibeta_p/1, Scope20/2  "Ibeta^*"
  Add8/1 -> Ialpha_p/1, Scope20/1  "Iaplha^*"
  Gain/1 -> Divide2/2, Divide4/2
  Gain5/1 -> Divide1/2, Divide3/2

== system deteccao_erro_2014/EHA3/DSP/Subsystem3 ==
  Ialpha_p : Inport
  Ibeta_p : Inport  Port=2
  Fcn1 : Fcn  Expr=sqrt(2/3)*u(1)
  Fcn2 : Fcn  Expr=sqrt(2/3)*(-1/2*u(1)+sqrt(3)/2*u(2))
  Fcn3 : Fcn  Expr=sqrt(2/3)*(-1/2*u(1)-sqrt(3)/2*u(2))
  Mux2 : Mux  Inputs=2
  Mux3 : Mux  Inputs=2
  Mux5 : Mux  Inputs=2
  Scope14 : Scope  NumInputPorts=3
      settings: TimeRange=0.08  YMin=-4~-4.5~-2  YMax=4.5~4~4.5  SaveName=ScopeData32
  Ia_C : Outport
  Ib_C : Outport  Port=2
  Ic_C : Outport  Port=3
  wires:
  Ibeta_p/1 -> Mux2/2, Mux3/2, Mux5/2
  Ialpha_p/1 -> Mux5/1, Mux2/1, Mux3/1
  Mux2/1 -> Fcn1/1
  Fcn1/1 -> Ia_C/1, Scope14/1  "Ia_C"
  Mux3/1 -> Fcn2/1
  Fcn2/1 -> Ib_C/1, Scope14/2  "Ib_C"
  Mux5/1 -> Fcn3/1
  Fcn3/1 -> Scope14/3, Ic_C/1  "Ic_C"

== system deteccao_erro_2014/EHA3/DSP/TCT ==
  Va : Inport
  Vb : Inport  Port=2
  Vc : Inport  Port=3
  Demux7 : Demux  Outputs=3
  Gain1 : Gain  Gain=sqrt(2/3)
  Gain3 : Gain  Gain=[1/sqrt(2), 1/sqrt(2), 1/sqrt(2); 1, -1/2, -1/2; 0, sqrt(3)/2, -sqrt(3)/2]  Multiplication=Matrix(K*u)
  Mux2 : Mux  Inputs=3
  valpha : Outport
  vbeta : Outport  Port=2
  wires:
  Gain3/1 -> Demux7/1  "Valphabeta0"
  Gain1/1 -> Gain3/1
  Mux2/1 -> Gain1/1
  Va/1 -> Mux2/1
  Vb/1 -> Mux2/2
  Vc/1 -> Mux2/3
  Demux7/2 -> valpha/1
  Demux7/3 -> vbeta/1

== system deteccao_erro_2014/EHA3/DSP/Transformada Inversa de Clarke ==
  valpha' : Inport
  vbeta' : Inport  Port=2
  Demux6 : Demux  Outputs=3
  Fcn10 : Fcn  Expr=sqrt(2/3)*(-1/2*u(1)+sqrt(3)/2*u(2))
  Fcn11 : Fcn  Expr=sqrt(2/3)*(-1/2*u(1)-sqrt(3)/2*u(2))
  Fcn9 : Fcn  Expr=sqrt(2/3)*(u(1) + 0*u(2))
  Mux{3,5,8..9} (4 alike) : Mux  Inputs=2
  Scope23 : Scope  NumInputPorts=3
      settings: YMin=-200~-200~-200  YMax=200~200~200  SaveName=ScopeData28
  va' : Outport
  vb' : Outport  Port=2
  vc' : Outport  Port=3
  wires:
  Fcn10/1 -> vb'/1, Scope23/2  "vb'"
  Demux6/1 -> Mux9/1
  valpha'/1 -> Mux5/1, Mux8/1, Mux3/1
  vbeta'/1 -> Mux3/2, Mux5/2, Mux8/2
  Mux5/1 -> Fcn10/1
  Mux3/1 -> Fcn9/1
  Fcn11/1 -> vc'/1, Scope23/3  "vc'"
  Fcn9/1 -> va'/1, Mux9/2  "va'"
  Mux8/1 -> Fcn11/1
  [Vabc_S] -> Demux6/1
  Mux9/1 -> Scope23/1

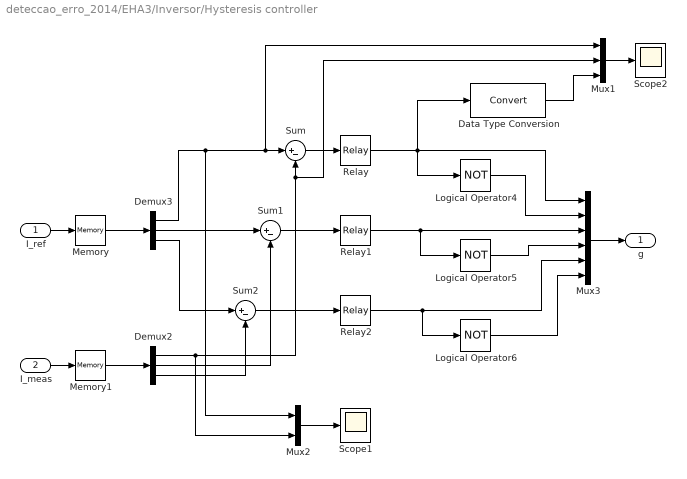
== system deteccao_erro_2014/EHA3/Inversor/Hysteresis controller ==
  I_ref : Inport
  I_meas : Inport  Port=2
  Data Type Conversion : DataTypeConversion
  Demux2 : Demux  Outputs=3
  Demux3 : Demux  Outputs=3
  Logical Operator4 : Logic  Operator=NOT  AllPortsSameDT=off  OutDataTypeStr=boolean
  Logical Operator5 : Logic  Operator=NOT  AllPortsSameDT=off  OutDataTypeStr=boolean
  Logical Operator6 : Logic  Operator=NOT  AllPortsSameDT=off  OutDataTypeStr=boolean
  Memory : Memory
  Memory1 : Memory
  Mux1 : Mux  Inputs=3
  Mux2 : Mux  Inputs=2
  Mux3 : Mux  Inputs=6
  Relay : Relay  OnSwitchValue=0.05  OffSwitchValue=-0.05  OutDataTypeStr=Inherit: Inherit via back propagation
  Relay1 : Relay  OnSwitchValue=0.05  OffSwitchValue=-0.05  OutDataTypeStr=Inherit: Inherit via back propagation
  Relay2 : Relay  OnSwitchValue=0.05  OffSwitchValue=-0.05  OutDataTypeStr=Inherit: Inherit via back propagation
  Scope1 : Scope
      settings: YMin=-3.75e+12  YMax=2.5e+11  SaveName=ScopeData30
  Scope2 : Scope
      settings: YMin=-4.5  YMax=5.5  SaveName=ScopeData6
  Sum : Sum  Inputs=|+-
  Sum1 : Sum  Inputs=|+-
  Sum2 : Sum  Inputs=|+-
  g : Outport
  wires:
  I_ref/1 -> Memory/1
  I_meas/1 -> Memory1/1
  Relay1/1 -> Logical Operator5/1, Mux3/3
  Demux3/1 -> Mux1/1, Sum/1, Mux2/1
  Logical Operator4/1 -> Mux3/2
  Logical Operator5/1 -> Mux3/4
  Logical Operator6/1 -> Mux3/6
  Mux3/1 -> g/1
  Demux2/1 -> Mux2/2, Mux1/2, Sum/2
  Memory/1 -> Demux3/1
  Memory1/1 -> Demux2/1
  Mux2/1 -> Scope1/1
  Sum/1 -> Relay/1
  Relay/1 -> Data Type Conversion/1, Mux3/1, Logical Operator4/1
  Demux3/2 -> Sum1/1
  Demux2/2 -> Sum1/2
  Sum1/1 -> Relay1/1
  Demux3/3 -> Sum2/1
  Sum2/1 -> Relay2/1
  Demux2/3 -> Sum2/2
  Relay2/1 -> Mux3/5, Logical Operator6/1
  Mux1/1 -> Scope2/1
  Data Type Conversion/1 -> Mux1/3

== system deteccao_erro_2014/EHA3/Inversor/PI controller ==
  Vdc : Inport
  Constant : Constant  Value=480
  LPF : dsparch4/Analog Filter Design  method=Butterworth  filttype=Lowpass  N=5  Wlo=2*pi*200  Whi=80  Rp=2  Rs=40
  PID Controller : simulink/Continuous/PID Controller  Controller=PI  TimeDomain=Continuous-time  SampleTime=-1  IntegratorMethod=Forward Euler  FilterMethod=Forward Euler  Form=Parallel  P=5  I=7  D=0  N=100  InitialConditionSource=internal  InitialConditionForIntegrator=0  InitialConditionForFilter=0  ExternalReset=none  LimitOutput=off  UpperSaturationLimit=inf  LowerSaturationLimit=-inf  LinearizeAsGain=on  AntiWindupMode=none  Kb=1  TrackingMode=off  Kt=1  PParamMin=[]  PParamMax=[]  IParamMin=[]  IParamMax=[]  DParamMin=[]  DParamMax=[]  NParamMin=[]  NParamMax=[]  KbParamMin=[]  KbParamMax=[]  KtParamMin=[]  KtParamMax=[]  POutMin=[]  POutMax=[]  IOutMin=[]  IOutMax=[]  DOutMin=[]  DOutMax=[]  NOutMin=[]  NOutMax=[]  KbOutMin=[]  KbOutMax=[]  KtOutMin=[]  KtOutMax=[]  IntegratorOutMin=[]  IntegratorOutMax=[]  FilterOutMin=[]  FilterOutMax=[]  SumOutMin=[]  SumOutMax=[]  SumI1OutMin=[]  SumI1OutMax=[]  SumI2OutMin=[]  SumI2OutMax=[]  SumI3OutMin=[]  SumI3OutMax=[]  SumDOutMin=[]  SumDOutMax=[]  SaturationOutMin=[]  SaturationOutMax=[]  IntegratorContinuousStateAttributes=''  IntegratorStateMustResolveToSignalObject=off  IntegratorRTWStateStorageClass=Auto  FilterContinuousStateAttributes=''  FilterStateMustResolveToSignalObject=off  FilterRTWStateStorageClass=Auto  DifferentiatorICPrevScaledInput=0  DifferentiatorOutMin=[]  DifferentiatorOutMax=[]  UseFilter=on
  Scope1 : Scope  NumInputPorts=2
      settings: TimeRange=0.015  YMin=372.5~72.5  YMax=407.5~107.5  SaveName=psb3phPWM1_str1  MaxDataPoints=500000
  Sum : Sum  Inputs=|-+
  Ploss : Outport
  wires:
  Vdc/1 -> Scope1/1, Sum/1
  Sum/1 -> Scope1/2, LPF/1
  Constant/1 -> Sum/2
  PID Controller/1 -> Ploss/1
  LPF/1 -> PID Controller/1

== system deteccao_erro_2014/EHA1/Inversor/PI controller/Signal Builder ==
  Demux : Demux  Tag=STV Demux  Outputs=1
  FromWs : FromWorkspace  Tag=STV FromWs  VariableName=tuvar  SampleTime=0
      SigBuilderData=|
      | common.afterFinalStr = 'Extrapolate'
      | common.sampleTime = 0
      | dataSet.timeRange = [72.8 73.9160839161]
      | dataSet.name = 'Imported_Group 1'
      | sbobj.Name = 'Signal Builder'
      | sbobj.Groups.Name = 'Imported_Group 1'
      | sbobj.Groups.Signals.Name = 'Signal 2'
      | sbobj.Groups.Signals.XData = [72.8 73.71 73.71 73.9160839161]
      | sbobj.Groups.Signals.YData = [0 0 620 620]
      | sbobj.Groups.TimeRange = [72.8 73.9160839161]
  Signal 2 : Outport  Tag=STV Outport
  wires:
  FromWs/1 -> Demux/1
  Demux/1 -> Signal 2/1
